simulink model "CvtRgbToGray"  (Simulink 7.1)
settings: Solver=VariableStepDiscrete  StartTime=0.0  StopTime=10  RelTol=1e-3
undefined symbols (not defined in the file): gray
libraries: vipsnks x2, vipsrcs x1
settings Model: Creator=lipingke  LastModifiedBy=lipingke

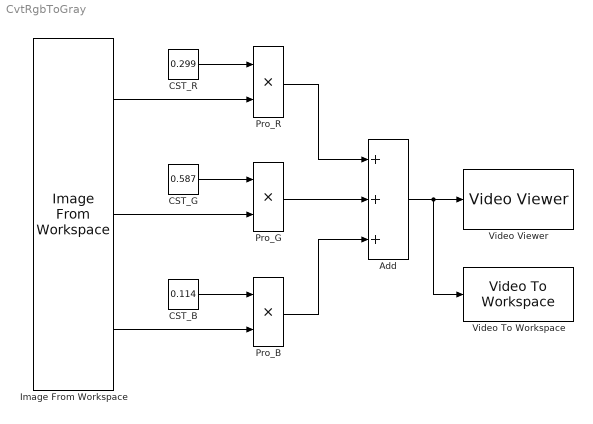
== system CvtRgbToGray ==
  Add : Sum  Inputs=+++  OutDataTypeMode=uint8  OutDataType=sfix(16)  OutScaling=2^-10  OutDataTypeStr=uint8
  CST_B : Constant  Value=0.114  OutDataType=sfix(16)  OutScaling=2^0
  CST_G : Constant  Value=0.587  OutDataType=sfix(16)  OutScaling=2^0
  CST_R : Constant  Value=0.299  OutDataType=sfix(16)  OutScaling=2^0
  Image From Workspace : vipsrcs/Image From Workspace  Tag=vipblks_nd  SystemSampleTime=-1  ImageValue=img  Ts=10  imagePorts=Separate color signals  ImageDataType=Inherit from 'Value'  Signed=on  WordLength=16  sdImageDataType=sfix(16)  FractionLengthMode=User-defined  FractionLength=15  OutPortLabels=R|G|B
  Pro_B : Product  OutDataType=sfix(16)  OutScaling=2^0  RndMeth=Zero
  Pro_G : Product  OutDataType=sfix(16)  OutScaling=2^0  RndMeth=Zero
  Pro_R : Product  OutDataType=sfix(16)  OutScaling=2^0  RndMeth=Zero
  Video To Workspace : vipsnks/Video To Workspace  DialogController=vipDDGCreate  DialogControllerArgs=DataTag0  VariableName=grayImg  NumInputs=1  DataLimit=10  DecimationFactor=1  LogFi=off  InPortLabels=R|G|B
  Video Viewer : vipsnks/Video Viewer  DialogController=vipDDGCreate  DialogControllerArgs=DataTag1  inputType=Obsolete7b  imagePorts=One multidimensional signal  useColorMap=off  colormapValue=gray(256)  specRange=off  minInputVal=0  maxInputVal=255  FigPos=[514 540 500 375]  AxisZoom=on  trueSizedOnce=on
  wires:
  CST_R/1 -> Pro_R/1
  Image From Workspace/3 -> Pro_B/2
  Image From Workspace/2 -> Pro_G/2
  CST_G/1 -> Pro_G/1
  CST_B/1 -> Pro_B/1
  Pro_G/1 -> Add/2
  Pro_R/1 -> Add/1
  Pro_B/1 -> Add/3
  Add/1 -> Video Viewer/1, Video To Workspace/1
  Image From Workspace/1 -> Pro_R/2
